simulink model "Question8"  (R2020a)
settings: Solver=VariableStepAuto  StartTime=0.0  StopTime=inf  RelTol=1e-3
undefined symbols (not defined in the file): allCarIds
libraries: sf_elevator_lib x2, sf_gui_elevator_controller_lib x2
settings Model: Creator=aishw  LastModifiedBy=aishw

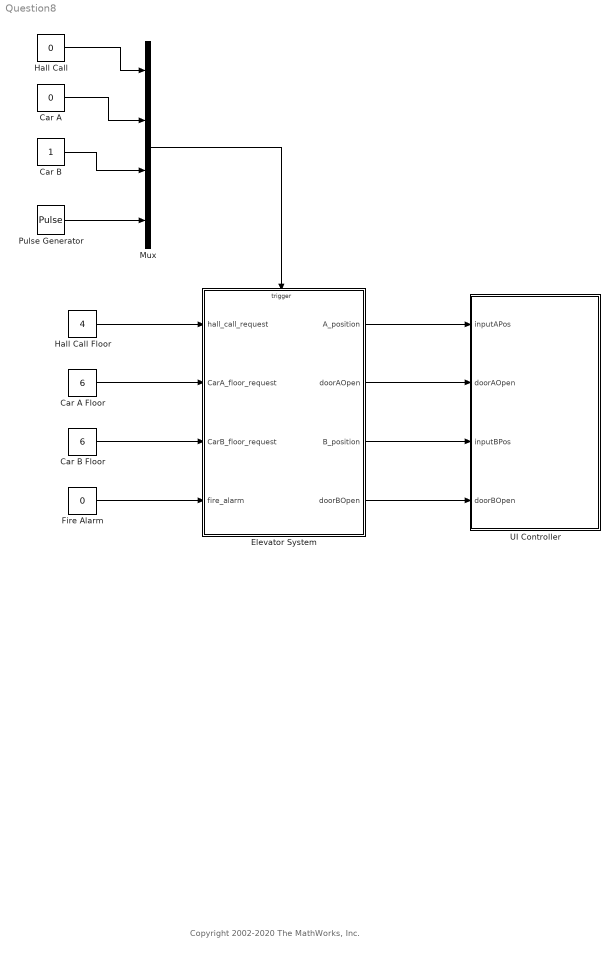
== system Question8 ==
  note: Copyright 2002-2020 The MathWorks, Inc.
  Car A : Constant  Value=0  OutDataTypeStr=double
  Car A Floor : Constant  Value=6  OutDataTypeStr=uint8
  Car B : Constant  OutDataTypeStr=double
  Car B Floor : Constant  Value=6  OutDataTypeStr=uint8
  Elevator System : Stateflow chart  TreatAsAtomicUnit=on
  Fire Alarm : Constant  Value=0  OutDataTypeStr=boolean
  Hall Call : Constant  Value=0  OutDataTypeStr=double
  Hall Call Floor : Constant  Value=4  OutDataTypeStr=uint8
  Mux : Mux
  Pulse Generator : DiscretePulseGenerator  PulseType=Time based  PulseWidth=50
  UI Controller : Stateflow chart  TreatAsAtomicUnit=on
  wires:
  Pulse Generator/1 -> Mux/4
  Car B/1 -> Mux/3
  Car A/1 -> Mux/2
  Hall Call/1 -> Mux/1
  Fire Alarm/1 -> Elevator System/4(fire_alarm)
  Elevator System/3(B_position) -> UI Controller/3(inputBPos)
  Hall Call Floor/1 -> Elevator System/1(hall_call_request)
  Elevator System/2(doorAOpen) -> UI Controller/2(doorAOpen)
  Mux/1 -> Elevator System/Trigger
  Car B Floor/1 -> Elevator System/3(CarB_floor_request)
  Car A Floor/1 -> Elevator System/2(CarA_floor_request)
  Elevator System/4(doorBOpen) -> UI Controller/4(doorBOpen)
  Elevator System/1(A_position) -> UI Controller/1(inputAPos)

== stateflow chart Question8/Elevator System ==
  state Elevator_Manager [parallel]
    settings: executionOrder=1
    state register(hall_call_floor) [function]
      (default) -> (junction 2062) : {enqueue(hall_call_floor);
          | hall_call_status[hall_call_floor] = 1;}
    state enqueue(hall_call_floor) [function]
      (default) -> (junction 1513)
      (junction 1513) -> (junction 1514) [order 1] : [hall_call_status[hall_call_floor] != 0]
      (junction 1513) -> (junction 1516) [order 2] : {i = 0;}
      (junction 1516) -> (junction 1515) [order 1] : [hall_call_queue[i] == hall_call_floor]
      (junction 1516) -> (junction 1516) [order 2] : [hall_call_queue[i] > 0 && i<NUM_FLOOR]{i++;}
      (junction 1516) -> (junction 1517) [order 3]
      (junction 1517) -> (junction 1518) [order 1] : [i >= NUM_FLOOR]
      (junction 1517) -> (junction 1519) [order 2] : {hall_call_queue[i] = hall_call_floor;}
    state process_hall_call [function]
      (default) -> (junction 2135)
      (junction 2135) -> (junction 2137) : {
          | /* 'INIT':Initialization */
          | request_floor = hall_call_queue[0];
          | }
      (junction 2137) -> (junction 2139) : {
          | /* Fire alarm is on */
          | fire_alarm_on = (fire_alarm);
          | }
      (junction 2139) -> (junction 2141) : {
          | /* There is outstanding request */
          | request_outstanding = (request_floor > 0);
          | }
      (junction 2141) -> (junction 2143) : {
          | /* Elevator A is idle */
          | elevator_A_idle = (Elevator_A.get_status() == ElevatorStatus.IDLE);
          | }
      (junction 2143) -> (junction 2145) : {
          | /* Elevator B is idle */
          | elevator_B_idle = (Elevator_B.get_status() == ElevatorStatus.IDLE);
          | }
      (junction 2145) -> (junction 2147) : {
          | /* Elevator A is closer to request */
          | elevator_A_closer = (fabs(Elevator_A.get_position() - request_floor) <= fabs(Elevator_B.get_position() - request_floor));
          | }
      (junction 2147) -> (junction 2149) [order 1] : [fire_alarm_on]
      (junction 2149) -> (junction 2151) : {
          | /* 'EMR':Emergency */
          | Elevator_A.register(floor(Elevator_A.get_position()+Elevator_A.get_direction()/2));
          | Elevator_B.register(floor(Elevator_B.get_position()+Elevator_B.get_direction()/2));
          | }
      (junction 2147) -> (junction 2153) [order 2]
      (junction 2153) -> (junction 2155) [order 1] : [!request_outstanding]
      (junction 2155) -> (junction 2157) : {
          | /* 'NONE':Both elevators are busy, OR no request present */
          |
          | }
      (junction 2153) -> (junction 2159) [order 2]
      (junction 2159) -> (junction 2161) [order 1] : [!elevator_A_idle && !elevator_B_idle]
      (junction 2161) -> (junction 2163) : {
          | /* 'NONE':Both elevators are busy, OR no request present */
          |
          | }
      (junction 2159) -> (junction 2165) [order 2]
      (junction 2165) -> (junction 2167) [order 1] : [elevator_A_idle && !elevator_B_idle]
      (junction 2167) -> (junction 2169) : {
          | /* 'A':Elevator A should respond to request */
          | Elevator_A.enqueue(request_floor);
          | Main_dequeue(request_floor);
          | }
      (junction 2165) -> (junction 2171) [order 2]
      (junction 2171) -> (junction 2173) [order 1] : [!elevator_A_idle && elevator_B_idle]
      (junction 2173) -> (junction 2175) : {
          | /* 'B':Elevator B should respond to request */
          | Elevator_B.enqueue(request_floor);
          | Main_dequeue(request_floor);
          | }
      (junction 2171) -> (junction 2177) [order 2]
      (junction 2177) -> (junction 2179) [order 1] : [elevator_A_idle && elevator_B_idle && elevator_A_closer]
      (junction 2179) -> (junction 2181) : {
          | /* 'A':Elevator A should respond to request */
          | Elevator_A.enqueue(request_floor);
          | Main_dequeue(request_floor);
          | }
      (junction 2177) -> (junction 2183) [order 2]
      (junction 2183) -> (junction 2185) : [elevator_A_idle && elevator_B_idle && !elevator_A_closer]
      (junction 2185) -> (junction 2187) : {
          | /* 'B':Elevator B should respond to request */
          | Elevator_B.enqueue(request_floor);
          | Main_dequeue(request_floor);
          | }
    Elevator_Manager -> (junction 2054) [order 1] : HALL_CALL {register(hall_call_request);}
    Elevator_Manager -> (junction 2057) [order 2] : CLOCK {process_hall_call();} //Clock drives whole system
  state result = Main_exists_in_queue(floor) [function]
    (default) -> (junction 1904) : {i=0;}
    (junction 1904) -> (junction 1904) [order 1] : [hall_call_queue[i] > 0 && ...
        | i<NUM_FLOOR && ...
        | hall_call_queue[i] != floor]{i++;}
    (junction 1904) -> (junction 1905) [order 2]
    (junction 1905) -> (junction 1906) [order 1] : [i >= NUM_FLOOR || hall_call_queue[i] == 0]{result = 0;}
    (junction 1905) -> (junction 1907) [order 2] : {result = i+1;}
  state Main_deregister(hall_call_floor) [function]
    (default) -> (junction 1898) : {Main_dequeue(hall_call_floor);
        | hall_call_status[hall_call_floor] = 0;}
  state Elevator_A [parallel]
    settings: executionOrder=2
  state Main_dequeue(hall_call_floor) [function]
    (default) -> (junction 1916) : {i=0;}
    (junction 1916) -> (junction 1916) [order 1] : [hall_call_queue[i] > 0 && ...
        | i<NUM_FLOOR && ...
        | hall_call_queue[i] != hall_call_floor]{i++;}
    (junction 1916) -> (junction 1917) [order 2]
    (junction 1917) -> (junction 1918) [order 1] : [i >= NUM_FLOOR || hall_call_queue[i] == 0]
    (junction 1917) -> (junction 1919) [order 2]
    (junction 1919) -> (junction 1920) : {hall_call_queue[i] = hall_call_queue[i+1]; i++;}
    (junction 1920) -> (junction 1919) [order 1] : [i < NUM_FLOOR]
    (junction 1920) -> (junction 1921) [order 2]
  state Elevator_B [parallel]
    settings: executionOrder=3
  data: hall_call_floor function_input double; hall_call_floor function_input uint8; i temporary uint8; request_floor temporary uint8; fire_alarm_on temporary boolean =0; request_outstanding temporary boolean =0; elevator_A_idle temporary boolean =0; elevator_B_idle temporary boolean =0; elevator_A_closer temporary boolean =0; result function_output uint8; floor function_input uint8; i temporary uint8; hall_call_floor function_input uint8; i temporary uint8; hall_call_floor function_input uint8; hall_call_request input uint8; A_position output double =6; NUM_FLOOR constant uint8 =5; CarA_floor_request input uint8; CarB_floor_request input uint8; fire_alarm input boolean; hall_call_queue local uint8 size=10; hall_call_status local uint8 size=10; doorAOpen output boolean =0; B_position output double =1; doorBOpen output boolean =0
  data fire_alarm_on settings: description=Fire alarm is on
  data request_outstanding settings: description=There is outstanding request
  data elevator_A_idle settings: description=Elevator A is idle
  data elevator_B_idle settings: description=Elevator B is idle
  data elevator_A_closer settings: description=Elevator A is closer to request
  events: HALL_CALL input EITHER_EDGE_EVENT; CAR_CALL_A input EITHER_EDGE_EVENT; CAR_CALL_B input EITHER_EDGE_EVENT; CLOCK input EITHER_EDGE_EVENT

== stateflow chart Question8/UI Controller ==
  state CarA_Controller [parallel]
    settings: executionOrder=1
  state CarB_Controller [parallel]
    settings: executionOrder=2
  data: inputAPos input; doorAOpen input; inputBPos input; doorBOpen input; allCarIds parameter uint8 size=2
